simulink model "simulation_outer_old"  (R2021b)
settings: Solver=VariableStepAuto  StartTime=0.0  StopTime=10.0  FixedStep=1e-6  RelTol=1e-3
settings Model: Creator=lab01  LastModifiedBy=joelm
settings SolverCC: AlgebraicLoopSolver=TrustRegion
settings DebuggingCC: SFMachineParentedDataDiag=warning

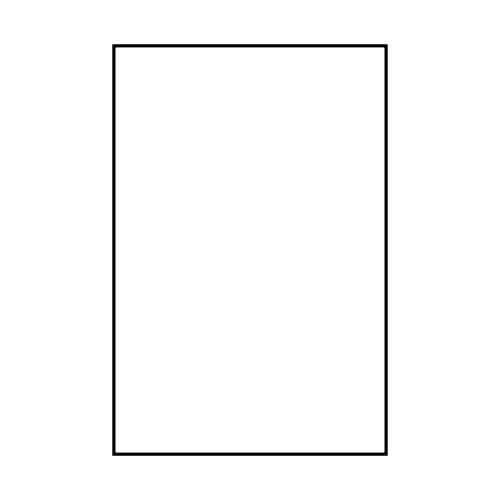
[thumbnail: Simulink's stored preview of the top-level diagram]
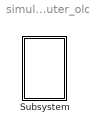
== system simulation_outer_old ==
  Subsystem : Subsystem

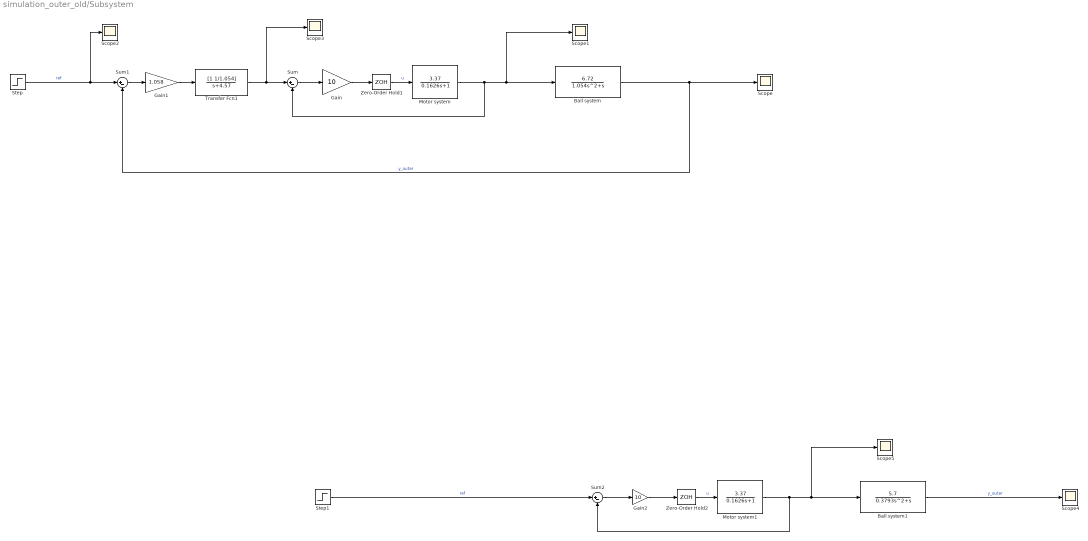
== system simulation_outer_old/Subsystem ==
  " Ball system" : TransferFcn  Numerator=[6.72]  Denominator=[1.054 1 0]
  " Ball system1" : TransferFcn  Numerator=[5.7]  Denominator=[0.3793 1 0]
  Gain : Gain  Gain=10
  Gain1 : Gain  Gain=1.058
  Gain2 : Gain  Gain=10
  Motor system : TransferFcn  Numerator=[0 3.37]  Denominator=[0.1626 1]
  Motor system1 : TransferFcn  Numerator=[0 3.37]  Denominator=[0.1626 1]
  Scope{,1..5} (6 alike) : Scope
  Step : Step
  Step1 : Step
  Sum : Sum  Inputs=|+-
  Sum1 : Sum  Inputs=|+-
  Sum2 : Sum  Inputs=|+-
  Transfer Fcn1 : TransferFcn  Numerator=[1 1/1.054]  Denominator=[1 4.57]
  Zero-Order Hold1 : ZeroOrderHold  SampleTime=0.005
  Zero-Order Hold2 : ZeroOrderHold  SampleTime=0.005
  wires:
  Step/1 -> Sum1/1, Scope2/1  "ref"
  Sum/1 -> Gain/1
  Gain/1 -> Zero-Order Hold1/1
  Zero-Order Hold1/1 -> Motor system/1  "u"
  Motor system/1 -> Sum/2, Scope1/1, " Ball system"/1
  " Ball system"/1 -> Scope/1, Sum1/2  "y_outer"
  Transfer Fcn1/1 -> Sum/1, Scope3/1
  Sum1/1 -> Gain1/1
  Gain1/1 -> Transfer Fcn1/1
  " Ball system1"/1 -> Scope4/1  "y_outer"
  Motor system1/1 -> Sum2/2, Scope5/1, " Ball system1"/1
  Gain2/1 -> Zero-Order Hold2/1
  Zero-Order Hold2/1 -> Motor system1/1  "u"
  Sum2/1 -> Gain2/1
  Step1/1 -> Sum2/1  "ref"
